simulink model "SimulArmV3"  (R2025b)
settings: Solver=VariableStepAuto  StartTime=0.0  StopTime=100  RelTol=1e-3  AbsTol=1e-3  EnableMultiTasking=on
values from neighbouring files (symbols this model uses):
  N = numel(data.t_ms_full)    [ServoStreamerTabbedUI.m]    (also in ServoStreamerUI.m; ServoStreamerUIV2.m; ServoStreamerUIV3.m; ServoStreamerUIV4.m)
  s = string(rx)    [ServoStreamerTabbedUI.m]    (also in ServoStreamerUI.m; ServoStreamerUIV6.m; ServoStreamerUIV7.m)
undefined symbols (not defined in the file or in its folder): X, Y, Z
libraries: sm_lib x45, nesl_utility x24, aerolibconvert2 x5, simulink x1
(part 1 of 3)
settings Model: SimulationMode=accelerator  Creator=ricky  LastModifiedBy=ricky
settings SolverCC: AutoScaleAbsTol=off  AlgebraicLoopSolver=TrustRegion  MaxZcPerStep=1.0
settings DataIOCC: LimitDataPoints=on  MaxDataPoints=10000
settings OptimizationCC: ReuseModelBlockBuffer=off  LifeSpan=inf
settings DebuggingCC: UnconnectedInputMsg=warning  UnconnectedOutputMsg=warning  UnconnectedLineMsg=warning  AllowSymbolicDim=off  SubsystemReferenceDiagnosticForUnitTest=warning  SFUnexpectedBacktrackingDiag=warning  SFNoUnconditionalDefaultTransitionDiag=warning  SFExecutionAtInitializationDiag=none  ArithmeticOperatorsInVariantConditions=warning
settings ModelReferenceCC: EnableRefExpFcnMdlSchedulingChecks=on
settings SFSimCC: SimUseLocalCustomCode=off  CustomCodeUndefinedFunction=UseInterfaceOnly
settings RTWCC: RTWUseLocalCustomCode=off  GPUComputeCapability=3.5  DLArmComputeVersion=19.05
settings CodeAppCC: StateflowObjectComments=on
settings GRTTargetCC: TargetLangStandard=C89/C90 (ANSI)
settings ConfigComp: CovMetricSettings=dw  CovSaveCumulativeToWorkspaceVar=on  CovSaveSingleToWorkspaceVar=on  CovExternalEMLEnable=off  CovSFcnEnable=off
settings SimscapeCC: SimscapeLogType=all  SimscapeLogSimulationStatistics=on  SimscapeLogDataHistory=10000.0

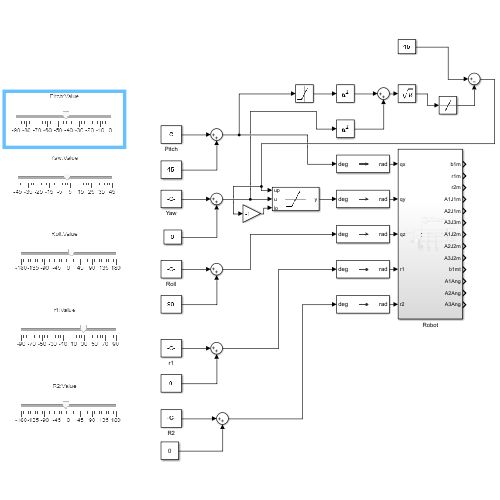
[thumbnail: Simulink's stored preview of the top-level diagram]
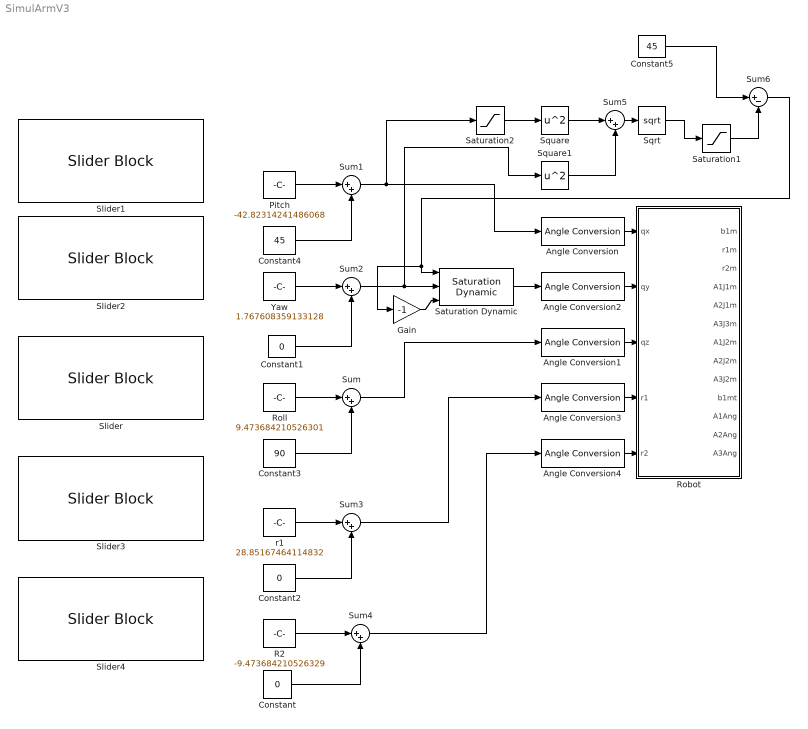
== system SimulArmV3 ==
  Angle Conversion{,1..4} (5 alike) : aerolibconvert2/Angle Conversion  IU=deg  OU=rad
  Constant : Constant  Value=0
  Constant1 : Constant  Value=0
  Constant2 : Constant  Value=0
  Constant3 : Constant  Value=90
  Constant4 : Constant  Value=45
  Constant5 : Constant  Value=45
  Gain : Gain  Gain=-1
  Pitch : Constant  Value=-42.82314241486068
  R2 : Constant  Value=-9.473684210526329
  Robot : Subsystem
  Roll : Constant  Value=9.473684210526301
  Saturation Dynamic : simulink/Discontinuities/Saturation Dynamic  OutMin=[]  OutMax=[]  OutDataTypeStr=Inherit: Same as second input  OutDataType=fixdt(1, 16)  OutScaling=2^-10  DoSatur=off
  Saturation1 : Saturate  UpperLimit=45  LowerLimit=0
  Saturation2 : Saturate  UpperLimit=45  LowerLimit=-45
  Slider : SliderBlock  ScaleMin=-180  ScaleMax=180
  Slider1 : SliderBlock  ScaleMin=-90  ScaleMax=0
  Slider2 : SliderBlock  ScaleMin=-45  ScaleMax=45
  Slider3 : SliderBlock  ScaleMin=-90  ScaleMax=90
  Slider4 : SliderBlock  ScaleMin=-180  ScaleMax=180
  Sqrt : Sqrt
  Square : Math  Operator=square
  Square1 : Math  Operator=square
  Sum{,1..5} (6 alike) : Sum  Inputs=|++
  Sum6 : Sum  Inputs=|+-
  Yaw : Constant  Value=1.767608359133128
  r1 : Constant  Value=28.85167464114832
  wires:
  Angle Conversion/1 -> Robot/1(qx)
  Angle Conversion1/1 -> Robot/3(qz)
  Sum/1 -> Angle Conversion1/1
  Constant3/1 -> Sum/2
  Sum1/1 -> Saturation2/1, Angle Conversion/1
  Constant4/1 -> Sum1/2
  Constant1/1 -> Sum2/2
  Angle Conversion2/1 -> Robot/2(qy)
  Roll/1 -> Sum/1
  Angle Conversion3/1 -> Robot/4(r1)
  Angle Conversion4/1 -> Robot/5(r2)
  r1/1 -> Sum3/1
  Constant2/1 -> Sum3/2
  R2/1 -> Sum4/1
  Constant/1 -> Sum4/2
  Sum3/1 -> Angle Conversion3/1
  Sum4/1 -> Angle Conversion4/1
  Pitch/1 -> Sum1/1
  Yaw/1 -> Sum2/1
  Square/1 -> Sum5/1
  Square1/1 -> Sum5/2
  Sum5/1 -> Sqrt/1
  Constant5/1 -> Sum6/1
  Sum6/1 -> Gain/1, Saturation Dynamic/1
  Gain/1 -> Saturation Dynamic/3
  Saturation Dynamic/1 -> Angle Conversion2/1
  Sqrt/1 -> Saturation1/1
  Sum2/1 -> Square1/1, Saturation Dynamic/2
  Saturation2/1 -> Square/1
  Saturation1/1 -> Sum6/2
